simulink model "valve_liquid_test"  (R2017b)
settings: Solver=VariableStepAuto  StartTime=0.0  StopTime=0  RelTol=1e-3
undefined symbols (not defined in the file or in its folder): CoolProp
libraries: thermochemical x2
settings Model: Creator=fferrucc  LastModifiedBy=fferrucc

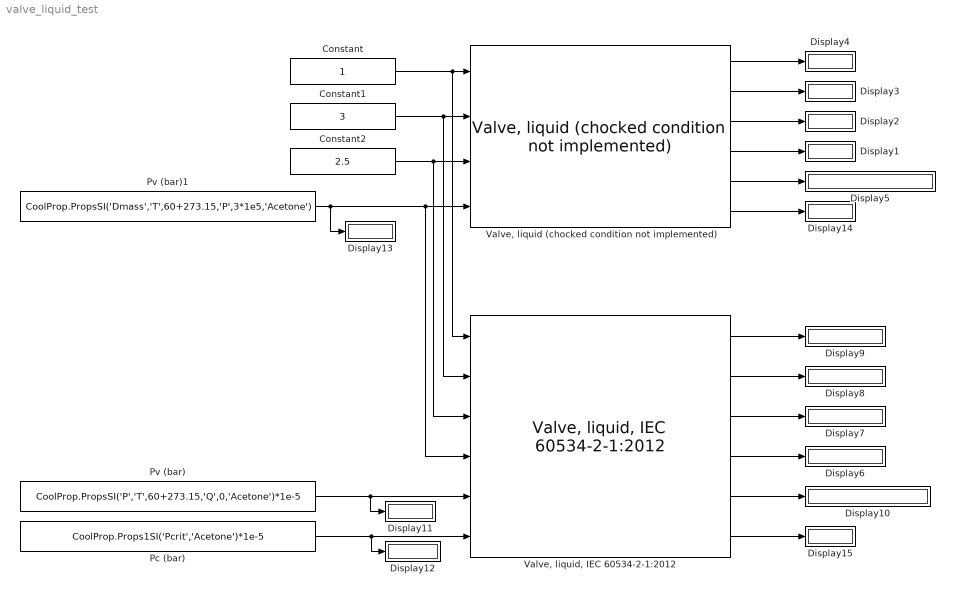
== system valve_liquid_test ==
  Constant : Constant
  Constant1 : Constant  Value=3
  Constant2 : Constant  Value=2.5
  Display{1..15} (15 alike) : Display
  Pc (bar) : Constant  Value=CoolProp.Props1SI('Pcrit','Acetone')*1e-5
  Pv (bar) : Constant  Value=CoolProp.PropsSI('P','T',60+273.15,'Q',0,'Acetone')*1e-5
  Pv (bar)1 : Constant  Value=CoolProp.PropsSI('Dmass','T',60+273.15,'P',3*1e5,'Acetone')
  "Valve, liquid (chocked condition not implemented)" : thermochemical/Valves/Valve, liquid (chocked condition not implemented)  Cv_dataPoints=[0 0.2 0.4 0.6 0.8 1]*1.0  apperture_dataPoints=[0 0.2 0.4 0.6 0.8 1]
      settings: SourceProductName=@ Thermochemical
  "Valve, liquid, IEC 60534-2-1:2012" : thermochemical/Valves/Valve, liquid, IEC 60534-2-1:2012  Cv_dataPoints=[0 0.2 0.4 0.6 0.8 1]*1.0  apperture_dataPoints=[0 0.2 0.4 0.6 0.8 1]  FL=0.74
      settings: SourceProductName=@ Thermochemical
  wires:
  "Valve, liquid (chocked condition not implemented)"/5 -> Display5/1
  "Valve, liquid (chocked condition not implemented)"/1 -> Display4/1
  "Valve, liquid (chocked condition not implemented)"/2 -> Display3/1
  "Valve, liquid (chocked condition not implemented)"/3 -> Display2/1
  "Valve, liquid (chocked condition not implemented)"/4 -> Display1/1
  Constant/1 -> "Valve, liquid (chocked condition not implemented)"/1, "Valve, liquid, IEC 60534-2-1:2012"/1
  Constant2/1 -> "Valve, liquid (chocked condition not implemented)"/3, "Valve, liquid, IEC 60534-2-1:2012"/3
  Constant1/1 -> "Valve, liquid (chocked condition not implemented)"/2, "Valve, liquid, IEC 60534-2-1:2012"/2
  Pv (bar)1/1 -> Display13/1, "Valve, liquid (chocked condition not implemented)"/4, "Valve, liquid, IEC 60534-2-1:2012"/4
  Pv (bar)/1 -> Display11/1, "Valve, liquid, IEC 60534-2-1:2012"/5
  Pc (bar)/1 -> Display12/1, "Valve, liquid, IEC 60534-2-1:2012"/6
  "Valve, liquid, IEC 60534-2-1:2012"/4 -> Display6/1
  "Valve, liquid, IEC 60534-2-1:2012"/3 -> Display7/1
  "Valve, liquid, IEC 60534-2-1:2012"/2 -> Display8/1
  "Valve, liquid, IEC 60534-2-1:2012"/1 -> Display9/1
  "Valve, liquid, IEC 60534-2-1:2012"/5 -> Display10/1
  "Valve, liquid (chocked condition not implemented)"/6 -> Display14/1
  "Valve, liquid, IEC 60534-2-1:2012"/6 -> Display15/1
